simulink model "MCLV_V2_33EP256MC506_SlidingModeObserver_Single_DualShunt"  (R2015b)
settings: Solver=FixedStepDiscrete  StartTime=0.0  StopTime=10.0  FixedStep=.00005  RelTol=1e-3
PreLoadFcn:
  | UserParams;
values from neighbouring files (symbols this model uses):
  DELTA_STARTUP_RAMP = round( (MINSPEEDINRPM*POLEPAIRS*LOOPTIMEINSEC*LOOPTIMEINSEC*65536*65536/(60*OPENLOOPTIMEINSEC)) )    [UserParams.m]
  TS = LOOPTIMEINSEC    (= 5e-05)    [UserParams.m]
undefined symbols (not defined in the file or in its folder): A4, C5, DiscIntNeverNeededParam, F1, Max, ms, P20, P53, P97, Pin, PWMmax, Resol, Timer, us
libraries: MCHP_Blockset x15, simulink x10, Lib_MCHP_BLKDEMO_Motor x2
settings Model: Creator=M91449  LastModifiedBy=M91449
settings OptimizationCC: DefaultParameterBehavior=Inlined  OptimizeModelRefInitCode=on  LifeSpan=1
settings HardwareCC: ProdBitPerInt=16  ProdBitPerPointer=32  ProdLargestAtomicInteger=Integer  ProdLargestAtomicFloat=None  ProdWordSize=16  ProdHWDeviceType=Generic->Custom
settings ModelReferenceCC: ModelReferenceNumInstancesAllowed=Single
settings RTWCC: SystemTargetFile=MCHP_dsPIC_stf.tlc  TemplateMakefile=MCHP_dsPIC.tmf  Description=Microchip Embedded Target PIC24 dsPIC30 dsPIC33 (real-time)  GenerateReport=on  IncludeHyperlinkInReport=on  LaunchReport=on  GenerateTraceInfo=on  GenerateTraceReport=on  GenerateTraceReportSl=on  GenerateTraceReportSf=on  GenerateTraceReportEml=on
settings CodeAppCC: IgnoreCustomStorageClasses=off  MaxIdLength=255
settings STFCustomTargetCC: TargetLibSuffix=_lib.a  ConcurrentExecutionCompliant=off  IncludeMdlTerminateFcn=off  GeneratePreprocessorConditionals=Use local settings  CombineOutputUpdateFcns=on  SuppressErrorStatus=on  ERTCustomFileBanners=on  SupportContinuousTime=off  MATLABClassNameForMDSCustomization=Simulink.SoftwareTarget.ERTCustomization  CPPClassGenCompliant=off  GRTInterface=off  SystemTargetFile=MCHP_dsPIC_stf.tlc
settings ERTTargetCC: TargetLibSuffix=_lib.a  ParMdlRefBuildCompliant=off  CompOptLevelCompliant=off  ConcurrentExecutionCompliant=off  IncludeMdlTerminateFcn=off  SuppressErrorStatus=on  ERTFirstTimeCompliant=off  SupportNonInlinedSFcns=on  ModelStepFunctionPrototypeControlCompliant=off  CPPClassGenCompliant=off  UseToolchainInfoCompliant=off  InlinedParameterPlacement=NonHierarchical  ERTSrcFileBannerTemplate=MCHP_dsPIC_code_template.cgt  ERTHdrFileBannerTemplate=MCHP_dsPIC_code_template.cgt  ERTDataSrcFileTemplate=MCHP_dsPIC_code_template.cgt  ERTDataHdrFileTemplate=MCHP_dsPIC_code_template.cgt  ERTCustomFileTemplate=MCHP_main.tlc

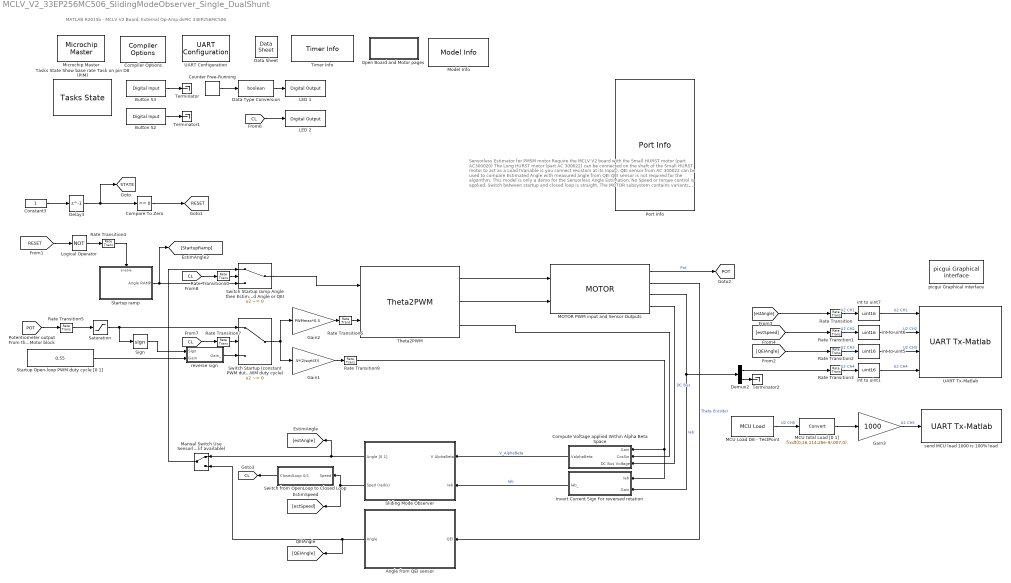
== system MCLV_V2_33EP256MC506_SlidingModeObserver_Single_DualShunt ==
  note: MATLAB R2015b - MCLV V2 Board, External Op-Amp dsPIC 33EP256MC506
  note: Sensorless Estimator for PMSM motor
      | Require the MCLV V2 board with the Small HURST motor (part AC300020)
      | The Long HURST motor (part AC 300022) can be connected on the shaft of the Small HURST motor
      | to act as a Load (Variable is you connect resistors at its Input).
      | QEI sensor from AC 300022 can be used to compare Estimated Angle with measured angle from QEI
      | QEI sensor is not required for the algorithm.
      |
      | This model is only a demo for the Sensorless Angle Estimation.
      | No Speed or torque control is applied. Switch between startup and closed loop is straight.
      |
      | The MOTOR subsystem contains variants. Right click on that MOTOR, and select
      | Dual Shunt or Single Shunt (edge aligned or center aligned) variants.
      | You might have to update the model twice after selecting a different variant.
      |
      | The Potentiometer were saturated to positive value only
      | as negative values does not work with Single Shunt Center Aligned for now
      |
      | MCU load is within 50% and 60% depending on Motor Variant selected.
      | Speed/Torque control loop might be executed at a lower rate than the model base rate (10kHz).
  Angle from QEI sensor : Subsystem
  Button S2 : MCHP_Blockset/Digital IO/Digital Input  PORT=Dynamic Options  PORT_TXT="G   [ 6 : 9 ]"  PIN=7  PACK=off  SIMULTANEOUS=off  ORDERING=None  SampleTime=.1  MCHP_PORT={Digital In}{DIN}2:0:G7;  MCHP_MASTERLINK=MCLV_V2_33EP256MC506_SlidingModeObserver_Single_DualShunt/Microchip Master
  Button S3 : MCHP_Blockset/Digital IO/Digital Input  PORT=Dynamic Options  PORT_TXT="G   [ 6 : 9 ]"  PIN=6  PACK=off  SIMULTANEOUS=off  ORDERING=None  SampleTime=.1  MCHP_PORT={Digital In}{DIN}2:0:G6;  MCHP_MASTERLINK=MCLV_V2_33EP256MC506_SlidingModeObserver_Single_DualShunt/Microchip Master
  Compare To Zero : simulink/Logic and Bit Operations/Compare To Zero  relop===  OutDataTypeStr=boolean
  Compiler Options : MCHP_Blockset/System Configuration/Compiler Options  Priority=1  LATEST_CMPLR=on  COMP_LIST=Dynamic Options  COMP_LIST_TXT=xc16 - v1.26  USE_64BIT_DOUBLE=off  MCHP_MULTITHREAD_COMPILATION=on  MCHP_MASTERLINK=MCLV_V2_33EP256MC506_SlidingModeObserver_Single_DualShunt/Microchip Master  OPTIMIZATION_LEVEL=3  MPLAB_LINKLIB=default  MPLAB_LINKLIB1=default  UNROLL_LOOPS=on  OMIT_FRAME_POINTER=off  PROCEDURAL_ABSTRACTION=off  MCONST=in code memory  MDATA=Use only memory below address 8192 (faster)  MSCALAR=Use only memory below address 8192 (faster)  MCODE=is less than 32768 (faster)  HEAP_SIZE=0  OMF=elf  DEBUG_INFO=off  AssemblyListing=on  ProduceHexOutput=off
  Compute Voltage applied Within Alpha Beta Space : Subsystem
  Constant3 : Constant  OutDataTypeStr=uint16  SampleTime=.1
  Counter Free-Running : simulink/Sources/Counter Free-Running  NumBits=1  tsamp=.1
  Data Sheet : MCHP_Blockset/System Info/Data Sheet  DOC_Type=datasheet  DOC_MCHP_Id=33EP256MC506_datasheet  DOC_FilePath=C:\Users\M91449\AppData\Local\Temp\70000657H.pdf  DOC_FileLastCheckTime="[2016              1             28             13             25         44.133]"  cpy_MCHP_Id=33EP256MC506  MCHP_MASTERLINK=MCLV_V2_33EP256MC506_SlidingModeObserver_Single_DualShunt/Microchip Master
      settings: AttributesFormatString=%<cpy_MCHP_Id>
  Data Type Conversion : DataTypeConversion  OutDataTypeStr=boolean
  Delay3 : Delay  DelayLength=1  InitialCondition=0
  Demux2 : Demux  Outputs=2
  Gain1 : Gain  Gain=.5*(2/sqrt(3))  OutDataTypeStr=fixdt(1,16,15)
  Gain2 : Gain  Gain=PWMmax*0.5  OutMin=-PWMmax*0.5  OutMax=PWMmax*0.5  OutDataTypeStr=fixdt(1,16)
  Gain3 : Gain  Gain=1000  OutDataTypeStr=uint16
  Invert Current Sign For reversed rotation : Subsystem
  LED 1 : MCHP_Blockset/Digital IO/Digital Output  PORT=Dynamic Options  PORT_TXT="D   [ 5  6  8 ]"  PIN=6  PACK=off  SIMULTANEOUS=off  READPREVIOUS=off  ORDERING=None  SampleTime=-1  MCHP_MASTERLINK=MCLV_V2_33EP256MC506_SlidingModeObserver_Single_DualShunt/Microchip Master
  LED 2 : MCHP_Blockset/Digital IO/Digital Output  PORT=Dynamic Options  PORT_TXT="D   [ 5  6  8 ]"  PIN=5  PACK=off  SIMULTANEOUS=off  READPREVIOUS=off  ORDERING=None  SampleTime=-1  MCHP_MASTERLINK=MCLV_V2_33EP256MC506_SlidingModeObserver_Single_DualShunt/Microchip Master
  Logical Operator : Logic  Operator=NOT  AllPortsSameDT=off  OutDataTypeStr=boolean
  MCU Load D8 - TestPoint : MCHP_Blockset/Profiling/MCU Load  MCULoadPin=Dynamic Options  MCULoadPin_TXT=None  MCULoadMeasure=on  TIMER_Resolution=Dynamic Options  TIMER_Resolution_TXT="Resol: 0.1143(us)  -  Max: 7.49(ms)"  MCHP_TIMER_REQUEST={MCU_Load}{MCU_Load}21:5:0:0:[]:524288;  MCHP_TIMER_RESULT=[2 65535 ]  MCHP_MASTERLINK=MCLV_V2_33EP256MC506_SlidingModeObserver_Single_DualShunt/Microchip Master  MCHP_COMPILED_INFO="CompiledSampleTime= [0.0070000000000000001   0 ];CompiledInportDataTypes=[ ];CompiledInportDataWidth=[];"  Info="Timer 2:  Resol: 114.2857143(ns)  -  Max: 7.48983(ms)"  SampleTime=.007
  MCU total Load [0 1] : DataTypeConversion  OutDataTypeStr=fixdt(0,16,114.28e-9/.007,0)  ConvertRealWorld=Stored Integer (SI)
  MOTOR PWM input and Sensor Outputs : Lib_MCHP_BLKDEMO_Motor/MOTOR  OverrideUsingVariant=(default)
  Manual Switch Use Sensorless Estimation or QEI (if available) : ManualSwitch
  Microchip Master : MCHP_Blockset/System Configuration/Microchip Master  Priority=1  PICREF=33EP256MC506  TIMESTEP_REF="Timer  ( 5e-05s )"  BUSYFLAG=Dynamic Options  BUSYFLAG_TXT=None  PWRTEN=PWRT enabled  BOREN=Disable  BODENV=2.7V  BORV=Brown-out Reset set at 2.0V  FPWRT=128ms  DSBOREN=Deep Sleep BOR enabled in Deep Sleep  DSLPBOR=Deep Sleep BOR enabled in Deep Sleep  MCLRE=RA5 input pin disabled;MCLR pin enabled  SMCLR=MCLR pin generates a normal system Reset  PMDL1WAY=Allow only one reconfiguration  RSTPRI=Device will obtain reset instruction from Primary flash  TEMP=Not used  SOSCSRC=Analog Mode for use with crystal  SOSCSEL=Secondary oscillator configured for high-power operation  IOL1WAY=Allow only one reconfiguration  ALTVREF=Voltage reference input; ADC =RA9/RA10 Comparator =RA9;RA10  DISUVREG=Regulator is disabled  DSSWEN=Deep Sleep is controlled by the register bit DSEN  LPCFG=Disabled - regardless of RETEN  RTCBAT=RTC operation is continued through VBAT  VBTBOR=VBAT BOR enabled  WUTSEL=Default regulator start-up time used  POWERSAVE=off  FNOSC=Primary oscillator (XT; HS; EC)  FPR=ECIO w/ PLL 16x  FOSFPR=HS3 w/PLL 16x  FOS=Primary Oscillator  FRANGE=High Range  OSCILLATOR_SELECT=Crystal / Ceramic resonator  OSCILLATOR_SELECT_spd=Crystal / Ceramic resonator  QUARTZ=8e6  QUARTZ_spd=8e6  POSCGAIN=2x gain setting  POSCBOOST=Boost the kick start of the oscillator  SOSCGAIN=2x gain setting  SOSCBOOST=Boost the kick start of the oscillator  ACTIV_PLL=on  ACTIV_PLL_spd=on  MIPS_DESIRED=70e6  MIPS_DESIRED_spd=70e6  FPLLMUL=24x Multiplier  FPLLIDIV=8x Divider  POSCFREQ=Primary oscillator/external clock input frequency greater than 8MHz  POSCMD=XT Crystal Oscillator Mode  POSCMOD=Primary Oscillator Disabled  MIPS=70 * 1e6  FPLLODIV=32x Divider  PLLKEN=Clock switch to PLL source will wait until the PLL lock signal is valid.  FCKSM=Both Clock Switching and Fail-safe Clock Monitor are enabled  FCKSMEN=Sw Disabled; Mon Disabled  IESO=Start up with FRC; then switch  DSWDTPS=1:2;147;483;648 (25.7 Days)  FWDTEN=Disable  FWDTWINSZ=Window size is 25%  FWPSA=WDT prescaler ratio of 1:128  FWPSA0=1:128  FWPSB=1:16  WDT=Disable  WDTPOST=1:32768  WDTPRE=1:128  WDTPS=1:32768  WINDIS=Watchdog Timer in Non-Window mode  WWDTEN=Non-Window mode  DSWDTEN=DSWDT enabled  DSWDTOSC=DSWDT uses Low Power RC Oscillator (LPRC)  FPBDIV=Pb_Clk is Sys_Clk/8  FSOSCEN=Enable SOSC  LPRCSEL=High Power; High Accuracy Mode  OSCIOFCN=OSCO/CLKO/RC15 functions as CLKO (FOSC/2)  OSCIOFNC=OSC2 is clock output  LVRCFG=Low Voltage regulator is not available  PLL_96MHZ=Enabled  PLL96MHZ=96 MHz PLL Startup is enabled automatically on start-up  PLLDIV=PLL is disabled  WDTCLK=WDT uses LPRC  WDTCMX=WDT clock source is determined by the WDTCLK Configuration bits  WDTWIN=WDT Window is 25% of WDT period  APL=Aux Flash Code protect is disabled  APLK=Aux Flash Write Protection or Code Protection is Enabled  AWRP=Auxiliary program memory is not write-protected  BSS=No boot program Flash segment  BWP=Protection Disabled  BWRP=Boot Segment may be written  CP=Protection Disabled  EBS=No Boot EEPROM  ESS=No Segment Data EEPROM  GCP=General Segment Code protect is disabled  GSS=General Segment Code protect is disabled  GSS0=No protection  GSSK=General Segment Write Protection or Code Protection is Enabled  GWRP=General Segment may be written  PWP=Disable  RBS=No Boot RAM  RSS=No Secure RAM  SSS=No Secure Segment  SWRP=Secure segment may be written  WPCFG=Disable  WPDIS=Disable  WPEND=Write Protect from WPFP to the last page of memory  WPFP=Page 127 (0x1FC00)  ICESEL=Communicate on PGEC1/PGED1  ICS=Communicate on PGEC2 and PGED2  JTAGEN=Disable  COE=Reset Into Operational Mode  RES=Not used  DEBUG=Debugger is disabled  BACKBUG=Not used  BKBUG=Device resets into Operational mode  ALTI2C=I2C mapped to SDA1/SCL1 pins  ALTI2C1=I2C1 mapped to SDA1/SCL1 pins  ALTI2C2=I2C2 mapped to SDA2/SCL2 pins  ALTQIO=QEA1; QEB1; INDX1 are selected as inputs to QEI1  ALTSS1=SS1A is selected as the I/O pin for SPI1  CMPPOL0=Hysteresis is applied to falling edge  CMPPOL1=Hysteresis is applied to falling edge  FCANIO=Default CAN I/O  FETHIO=Default Ethernet I/O  FMIIEN=MII Enabled  FSRSSEL=SRS Priority 7  FUSBIDIO=Controlled by the USB Module  FVBUSONIO=Controlled by USB Module  HPOL=PWM module high side output pins have active-high output polarity  HYST0=45 mV Hysteresis  HYST1=45 mV Hysteresis  I2C1SEL=Use Default SCL1/SDA1 Pins For I2C1  LPOL=PWM module low side output pins have active-high output polarity  PWMPIN=PWM module pins controlled by PORT register at device Reset  RTCOSC=RTCC uses Secondary Oscillator (SOSC)  UPLLEN=USB PLL is enabled  UPLLIDIV=12x Divider  ATMOD8=Not used  ALTPMP=EPMP pins are in default location mode  I2C2SEL=I2C2 is multiplexed to SDA2/RA3 and SCL2/RA2  ALTADREF=AVREF+/AVREF- are mapped to RA9/RA10  ALTCVREF=CVREF+/CVREF- are mapped to RA9/RA10  PWMLOCK=PWM registers may be written without key sequence  MCHP_TIMER_REQUEST={Time Step}{TS}0:2:3:1:[]:3500;  MCHP_TIMER_RESULT=[1 3498.9999999999991 ]  MCHP_PLLRegisters="[5    243  16385     -1]"  MCHPVAR=MCHP.fcy.periph=70000000;MCHP.fcy.MIPS=70000000;MCHP.PowerSave=0;MCHP.TimeStepFactor=MCHP_Fun.Hex2num('[3FF0000000000001]');MCHP.TimeStep_Timer=1;MCHP.NTIMERS=5;MCHP.id.name='33EP256MC506';MCHP.id.N=reshape([33 256 506],1,3);MCHP.id.L=reshape({ 'EP','MC',''},1,3);MCHP.id.Arch=3;MCHP.periph.PPS.reg_RPINRx=reshape([-1 1 1 -1 -1 -1 1 -1 -1 -1 -1 -1 -1 -1 1 1 1 1 -1 -1 -1 -1 -1 -1 1 1 -1 -1 1 1 1 1 -1 -1 -1 -1 1 -1 1 -1 -1 -1 -1 -1 1 1 1 -1 -1 -1 -1 -1 1 -1 -1 -1 -1 -1 -1 -1 -1 -1 -1 -1 -1 -1 -1 -1 -1 -1 -1 -1 -1 -1 -1 1 -1 1 1 1],1,80);MCHP.PPS.dsPIC.RP=reshape([-1 -1 -1 -1 -1 -1 -1 -1 -1 -1 -1 -1 -1 -1 -1 -1 -1 -1 -1 -1 4 -1 -1 -1 -1 -1 -1 -1 -1 -1 -1 -1 -1 -1 -1 19 20 21 22 23 24 25 26 27 -1 -1 -1 -1 -1 -1 -1 -1 -1 -1 38 39 40 41 -1 -1 -1 -1 -1 -1 -1 -1 -1 -1 -1 -1 -1 -1 -1 -1 -1 -1 -1 -1 -1 -1 -1 -1 -1 -1 -1 -1 -1 -1 -1 -1 -1 -1 -1 -1 -1 -1 -1 81 -1 -1 -1 -1 -1 -1 -1 -1 -1 -1 -1 -1 -1 -1 -1 -1 -1 -1 -1 -1 102 -1 104],1,121);MCHP.PPS.dsPIC.RPI=reshape([-1 -1 -1 -1 -1 -1 -1 -1 -1 -1 -1 -1 -1 -1 -1 -1 -1 -1 -1 -1 -1 -1 -1 -1 8 9 -1 11 12 -1 -1 -1 16 17 18 -1 -1 -1 -1 -1 -1 -1 -1 -1 28 29 30 31 -1 -1 -1 35 36 37 -1 -1 -1 -1 42 -1 -1 -1 -1 -1 -1 -1 -1 -1 -1 -1 -1 -1 -1 -1 -1 -1 -1 -1 -1 -1 -1 -1 -1 -1 -1 -1 -1 -1 -1 -1 -1 -1 -1 -1 78 79 80 -1 -1 -1 -1 -1 -1 -1 -1 -1 -1 -1 -1 -1 -1 -1 -1 -1 -1 -1 -1 -1 -1 103 -1 105],1,122);MCHP.PPS.dsPIC.RPINR_list=reshape({ '1','INT1','INT2','INT3','INT4','T1CK','T2CK','T3CK','T4CK','T5CK','T6CK','T7CK','T8CK','T9CK','IC1','IC2','IC3','IC4','IC5','IC6','IC7','IC8','OCFA','OCFB','FLT1','FLT2','FLT3','FLT4','QEA1','QEB1','INDX1','HOME1','QEA2','QEB2','INDX2','HOME2','U1RX','U1CTS','U2RX','U2CTS','SDI1','SCK1','SS1','44','SDI2','SCK2','SS2','48','CSDIR','CSCK','COFS','52','C1RX','C2RX','U3RX','U3CTS','U4RX','U4CTS','SDI3','SCK3','SS3','62','SDI4','SCK4','SS4','66','IC9','IC10','IC11','IC12','IC13','IC14','IC15','IC16','OCFC','SYNCI1','SYNCI2','DTCMP1','DTCMP2','DTCMP3','DTCMP4','DTCMP5','DTCMP6','DTCMP7','FLT5','FLT6','FLT7','FLT8','89','SENT1','SENT2','92'},1,92);MCHP.PPS.dsPIC.RPOR_list=reshape({ '1','U1TX','U1RTS','U2TX','U2RTS','SDO1','SCK1','SS1','SDO2','SCK2','SS2','CSDO','CSCK','COFS','C1TX','C2TX','OC1','OC2','OC3','OC4','OC5','OC6','OC7','OC8','C1OUT','C2OUT','C3OUT','U3TX','U3RTS','U4TX','U4RTS','SDO3','SCK3','SS3','SDO4','SCK4','SS4','OC9','OC10','OC11','OC12','OC13','OC14','OC15','OC16','SYNCO1','SYNCO2','QEI1CCMP','QEI2CCMP','REFCLK','C4OUT','C5OUT','52','53','54','55','56','SENT1','SENT2'},1,59);MCHP.PPS.map_RPnR_RPORx=reshape([20 35 36 37 38 39 40 41 42 43 54 55 56 57 -1 97 -1 118 120],1,19);MCHP.Rx=reshape([13 15 21 -1 -1 58 -1 -1 -1 -1 -1 14 16 22 -1 -1 59 -1 -1 -1 -1 -1 -1 17 23 -1 -1 -1 -1 -1 -1 -1 -1 -1 18 35 -1 -1 -1 -1 -1 -1 -1 -1 33 32 36 -1 -1 -1 -1 -1 -1 -1 -1 -1 43 37 53 -1 -1 -1 -1 -1 -1 -1 -1 44 50 54 -1 -1 4 -1 -1 -1 -1 1 46 51 -1 -1 -1 5 -1 -1 -1 -1 31 48 52 42 -1 -1 6 -1 -1 -1 -1 34 49 55 -1 -1 -1 8 -1 -1 -1 -1 64 60 45 -1 -1 -1 -1 -1 -1 -1 -1 12 61 24 -1 -1 -1 -1 -1 -1 -1 -1 11 62 39 -1 27 -1 -1 -1 -1 -1 -1 -1 63 47 -1 28 -1 -1 -1 -1 -1 -1 -1 2 -1 -1 29 -1 -1 -1 -1 -1 -1 -1 3 40 -1 30 -1 -1 -1 -1 -1 -1],11,16);MCHP.ADC.ANtype=reshape([3 0],1,2);MCHP.ADC.ADCONx=reshape([47103 59391 40959 263 0 0],1,6);MCHP.ADC.ADCHS_0=reshape([40863 1799],1,2);MCHP.ADC.Flags=reshape([1 0],1,2);MCHP.ADC.Buffer=reshape([16 -1],1,2);MCHP.ADC.port=reshape([0 1 16 17 18 19 32 33 34 11 12 43 76 77 78 79 -1 -1 -1 -1 -1 -1 -1 -1 -1 -1 -1 -1 -1 -1 -1 -1 -1 -1 -1 -1 -1 -1 -1 -1 -1 -1 -1 -1 -1 -1 -1 -1 -1 -1 -1 -1 -1 -1 -1 -1 -1],1,57);MCHP.ADC.port_VrefP=17;MCHP.ADC.port_VrefM=16;MCHP.ADC.port_AVdd=-1;MCHP.ADC.port_AVss=-1;MCHP.memory.RAM=32768;MCHP.memory.RAM_XBegin=4096;MCHP.memory.RAM_YBegin=20480;MCHP.memory.RAM_dma=reshape([-1 -1],1,2);MCHP.DMA.Num=4;MCHP.DMA.CNTmax=16383;MCHP.QEI.QEICONx=reshape([49023 -1 -1 -1 -1 -1],1,6);MCHP.QEI.QEItype=1;MCHP.QEI.Port_QEI_INDX=reshape([-1 -1],1,2);MCHP.QEI.Port_QEI_QEA=reshape([-1 -1],1,2);MCHP.QEI.Port_QEI_QEB=reshape([-1 -1],1,2);MCHP.QEI.Port_QEI_UPDN=reshape([-1 -1],1,2);MCHP.INT.Port=reshape([23 32767 32767 -1 -1],1,5);MCHP.PWM_HS.Flags=reshape([3 1 0],1,3);MCHP.PWM.port_FLT=reshape([-1 -1 -1 34 43 -1 -1 -1 -1 -1 -1 -1 -1 -1 -1 -1 -1 -1 -1 -1 -1 -1 -1 -1 -1 -1 -1 -1 -1 -1 -1 -1 20],1,33);MCHP.PWM.PWMRef=-1;MCHP.PWM.Flag=0;MCHP.PWM.Port_PWM_l=reshape([31 -1 29 -1 27 -1 -1 -1 -1 -1 -1 -1 -1 -1 -1 -1 -1 -1],2,9);MCHP.PWM.Port_PWM_h=reshape([30 -1 28 -1 26 -1 -1 -1 -1 -1 -1 -1 -1 -1 -1 -1 -1 -1],2,9);MCHP.IC.Port=reshape([32767 32767 32767 32767 0 0 0 0 0 0 0 0 0 0 0 0],1,16);MCHP.IC.type=1;MCHP.OC.Port=reshape([32767 32767 32767 32767 0 0 0 0 0 0 0 0 0 0 0 0],1,16);MCHP.OC.type=1;MCHP.CN.Port=reshape([-1 -1 -1 -1 -1 -1 -1 -1 -1 -1 -1 -1 -1 -1 -1 -1 -1 -1 -1 -1 -1 -1 -1 -1 -1 -1 -1 -1 -1 -1 -1 -1 -1 -1 -1 -1 -1 -1 -1 -1 -1 -1 -1 -1 -1 -1 -1 -1 -1 -1 -1 -1 -1 -1 -1 -1 -1 -1 -1 -1 -1 -1 -1 -1 -1 -1 -1 -1 -1 -1 -1 -1 -1 -1 -1 -1 -1 -1 -1 -1 -1 -1 -1 -1 -1],1,85);MCHP.CN.PullUp=reshape([8083 65535 49151 352 61440 3 960 0 0 0 0],1,11);MCHP.CN.type=1;MCHP.CN.Flag_PullDown=1;MCHP.SPI.Refs=reshape([1 2 0 0 0 0],1,6);MCHP.SPI.SPIxCON1=8191;MCHP.SPI.SPIxCON2=57347;MCHP.SPI.Port_SDI=reshape([9 -1 -1 -1 -1 -1],1,6);MCHP.SPI.Port_SDO=reshape([4 -1 -1 -1 -1 -1],1,6);MCHP.SPI.Port_SCK=reshape([35 -1 -1 -1 -1 -1],1,6);MCHP.SPI.Port_SS=reshape([16 -1 -1 -1 -1 -1],1,6);MCHP.I2C.Refs=reshape([1 2 0 0 0],1,5);MCHP.I2C.I2CxCON=49151;MCHP.I2C.NewRegName=1;MCHP.I2C.Port_SDA=reshape([36 8 -1 -1 -1],1,5);MCHP.I2C.Port_SCL=reshape([37 20 -1 -1 -1],1,5);MCHP.I2C.Port_ASDA=reshape([25 21 -1 -1 -1],1,5);MCHP.I2C.Port_ASCL=reshape([24 22 -1 -1 -1],1,5);MCHP.I2C.Fuse_Port_SCL_SDA=reshape([3 1 4 1 -1 -1 -1 -1 -1 -1],2,5);MCHP.I2C.Fuse_Port_ASCL_ASDA=reshape([3 2 4 2 -1 -1 -1 -1 -1 -1],2,5);MCHP.Comp.Port_CVrefin=-1;MCHP.Comp.Port_CVref=-1;MCHP.Comp.Port_CVref1O=24;MCHP.Comp.Port_CVref2O=4;MCHP.Comp.Port_CxOUT=reshape([32767 32767 32767 32767 -1],1,5);MCHP.Comp.Port_OAxOUT=reshape([17 0 32 -1 -1],1,5);MCHP.Comp.Port_CxINP=reshape([18 1 34 32 -1],1,5);MCHP.Comp.Port_CxINM=reshape([19 43 -1 -1 16 76 -1 -1 33 77 -1 -1 33 -1 -1 -1 -1 -1 -1 -1],4,5);MCHP.Comp.nComp=reshape([4 0 0],1,3);MCHP.Comp.OpAmp=7;MCHP.Comp.CVRCON=reshape([17663 0],1,2);MCHP.UART.port_Rx=reshape([32767 32767 -1 -1 -1 -1],1,6);MCHP.UART.port_Tx=reshape([32767 32767 -1 -1 -1 -1],1,6);MCHP.UART.port_ARx=reshape([-1 -1],1,2);MCHP.UART.port_ATx=reshape([-1 -1],1,2);MCHP.UART.port_RTS=reshape([34 76 -1 -1 -1 -1],1,6);MCHP.UART.port_CTS=reshape([43 77 -1 -1 -1 -1],1,6);MCHP.UART.reg_UxMODE=reshape([48127 48127 -1 -1 -1 -1],1,6);MCHP.UART.reg_UxSTA=reshape([61439 61439 -1 -1 -1 -1],1,6);  MCHP_CRC=2647204  BTMODE=Device is in Single Boot (legacy) mode  RES1=Not used  PLLSS=PLL is fed by the Primary oscillator  RES2=Not used  ALTCMPI=C1INC is on RB13; C2INC is on RB9 and C3INC is on RA0  BOREN1=BOR Enabled [When BOREN=1]  ALTRB6=Append the RP6/ASCL1/PMPD6 functions of RB6 to RA1 pin functions  RETCFG=Retention regulator is not available  DFMCY=Not used  BSS2=No Boot Segment  BSEN=No Boot Segment  CWRP=Configuration Segment may be written  CSS=No Protection (other than CWRP)  AIVTDIS=Disable Alternate Vector Table  BSLIM=Not used  WDTEN=Disable  BTSWP=Not used  DBCC=Not used  CTXT1=Not Assigned  CTXT2=Not Assigned  SEQNUM=Not used  nSEQNUM=Not used  BOREN0=Enabled  DMTIVT=Not used  DMTCNT=2^31 (2147483648)  DMTEN=Dead Man Timer is Disabled and can be enabled by software  ON=Not used  USERID=Not used  RESERVED1=Not used  PGL1WAY=Allow only one reconfiguration  FPLLRNG=34-68 MHz Input  FPLLICLK=FRC is input to the System PLL  FPLLMULT=PLL Multiply by 128  UPLLFSEL=USB PLL input is 24 MHz  DMTINTV=Window/Interval value is 127/128 counter value  WDTSPGM=WDT stops during Flash programming  FDMTEN=Deadman Timer is disabled  TRCEN=Trace features in the CPU are enabled  BOOTISA=Boot code and Exception code is MIPS32  FECCCON=ECC and Dynamic ECC are disabled (ECCCON bits are writable)  EXTDDRSIZE=External DDR2 Size is 128 MB  FSLEEP=Flash is powered down when the device is in Sleep mode  DBGPER=Allow CPU access to all permission regions  EJTAGBEN=Normal EJTAG functionality  TSEQ=Not used  CSEQ=Not used
  Model Info : simulink/Model-Wide Utilities/Model Info  Frame=on  DisplayStringWithTags=|  HorizontalTextAlignment=Left  LeftAlignmentValue=0.02  SourceBlockDiagram=MCLV_V2_33EP256MC506_SlidingModeObserver_Single_DualShunt  TagMaxNumber=20
      | Short hust motor with:
      | M1 - Black
      | M2 - Red
      | M3 - White
  Open Board and Motor pages : Subsystem
      settings: OpenFcn=|
      | web('www.microchip.com/DevelopmentTools/ProductDetails.aspx?PartNO=DM330021-2','-browser');
      | pause(1);
      | web('http://www.microchipdirect.com/productsearch.aspx?keywords=AC300020','-browser');
      | pause(1);
      | web('www.microchipdirect.com/ProductSearch.aspx?keywords=AC300022','-browser');
      mask Display: disp('Open tools\nWebpage');
  Port Info : MCHP_Blockset/System Info/Port Info  MCHP_MASTERLINK=MCLV_V2_33EP256MC506_SlidingModeObserver_Single_DualShunt/Microchip Master
  Rate Transition{,1..4,6..7,9..10} (9 alike) : RateTransition
  Rate Transition5 : RateTransition  OutPortSampleTime=.1
  Saturation : Saturate  UpperLimit=1  LowerLimit=0
  Sign : Signum
  Sliding Mode Observer : Subsystem
  Startup Open-loop PWM duty cycle [0 1] : Constant  Value=0.55  OutDataTypeStr=Inherit: Inherit via back propagation
  Startup ramp : Subsystem
  Switch Startup (constant PWM duty cycle) then Closed Loop (Pot drive PWM duty cycle) : Switch  Criteria=u2 ~= 0  Threshold=250
  Switch Startup ramp Angle then Estimated Angle or QEI : Switch  Criteria=u2 ~= 0  Threshold=250
  Switch from OpenLoop to Closed Loop : Subsystem
  Tasks State Show base rate Task on pin D8 (PIM) : MCHP_Blockset/Profiling/Tasks State  TasksPin=D8  MCHP_PORT={Task D1 Running}{Task D1}15:1:D8;  MCHP_MASTERLINK=MCLV_V2_33EP256MC506_SlidingModeObserver_Single_DualShunt/Microchip Master
  Terminator : Terminator
  Terminator1 : Terminator
  Terminator2 : Terminator
  Theta2PWM : Lib_MCHP_BLKDEMO_Motor/Theta2PWM  VariantControl=Variant  OverrideUsingVariant=Optimized
  Timer Info : MCHP_Blockset/System Info/Timer Info  MCHP_MASTERLINK=MCLV_V2_33EP256MC506_SlidingModeObserver_Single_DualShunt/Microchip Master
  UART Configuration : MCHP_Blockset/BUS UART/UART Configuration  UART_REF=2  BAUD_Choice=Dynamic Options  BAUD_Choice_TXT="921600         [-0.06%]"  BAUD_Choice_IR=Dynamic Options  BAUD_Choice_IR_TXT=[]  BAUD_Custom=115200  IRDA=off  ALT_IO=on  PIN_RX=Dynamic Options  PIN_RX_TXT=C5 / P53 / Pin[37]  PIN_TX=Dynamic Options  PIN_TX_TXT=F1 / P97 / Pin[59]  FlowControl=None  PIN_CTS=Dynamic Options  PIN_CTS_TXT=A4 / P20 / Pin[33]  PIN_RTS=Dynamic Options  PIN_RTS_TXT=A4 / P20 / Pin[33]  MCHP_PORT="{UART2  Rx}{U2RX}3:0:P53;{UART2  Tx}{U2TX}3:1:P97;"  MCHP_MASTERLINK=MCLV_V2_33EP256MC506_SlidingModeObserver_Single_DualShunt/Microchip Master  MCHP_COM_ExtPil=off  TX_IMPLEMENTATION=DMA Ping-Pong Mode  TX_INT_PRIORITY=2  TX_INT_WHEN=is empty & last char is sent  TX_CIRCULAR_SIZE=32  TX_DMA_CHANNEL="0   (Lowest Priority)"  TX_DMA_SIZE=60  RX_IMPLEMENTATION=Simplest (4 bytes internal buffer only)  RX_INT_PRIORITY=1  RX_INT_WHEN=receive 1 character  RX_CIRCULAR_SIZE=32  InitSequence_chkbox=off  BAUD_Choice_InitSeq=Dynamic Options  BAUD_Choice_InitSeq_TXT="110         [-0.00%]"  BAUD_Choice_IR_InitSeq=Dynamic Options  BAUD_Choice_IR_InitSeq_TXT=0  BAUD_Custom_InitSeq=0  InitSequence='Hello World'
  UART Tx-Matlab : MCHP_Blockset/BUS UART/UART Tx-Matlab  UART_REF=2  CHANNELS=[1 2 3 4]  AllOrNothing=on  SampleTime=.00015  MCHP_MASTERLINK=MCLV_V2_33EP256MC506_SlidingModeObserver_Single_DualShunt/Microchip Master  MCHP_COMPILED_INFO="CompiledSampleTime= [0.00014999999999999999   0 ];CompiledInportDataTypes=[  5   5   5   5 ];CompiledInportDataWidth=[1  1  1  1];"
  int to uint{1,5..7} (4 alike) : DataTypeConversion  OutDataTypeStr=uint16  ConvertRealWorld=Stored Integer (SI)
  picgui Graphical interface : MCHP_Blockset/BUS UART/picgui Graphical interface  Nothing=0
  reverse sign : Subsystem
  send MCU load 1000 is 100% load : MCHP_Blockset/BUS UART/UART Tx-Matlab  UART_REF=2  CHANNELS=5  AllOrNothing=on  SampleTime=-1  MCHP_MASTERLINK=MCLV_V2_33EP256MC506_SlidingModeObserver_Single_DualShunt/Microchip Master  MCHP_COMPILED_INFO="CompiledSampleTime= [0.0070000000000000001   0 ];CompiledInportDataTypes=[  5 ];CompiledInportDataWidth=[1];"
  tag scope: CL=global, POT=global, RESET=global, STATE=global
  wires:
  Counter Free-Running/1 -> Data Type Conversion/1
  Data Type Conversion/1 -> LED 1/1
  [CL] -> LED 2/1
  Rate Transition/1 -> int to uint7/1  "U2 CH1"
  Rate Transition1/1 -> int to uint6/1  "U2 CH2"
  MCU Load D8 - TestPoint/1 -> MCU total Load [0 1]/1  "U2 CH5"
  Constant3/1 -> Delay3/1
  Delay3/1 -> Compare To Zero/1, [STATE]
  Sliding Mode Observer/2(Sped (rad/s)) -> [estSpeed], Switch from OpenLoop to Closed Loop/1(Speed)
  Switch Startup ramp Angle then Estimated Angle or QEI/1 -> Theta2PWM/1
  [estAngle] -> Rate Transition/1
  [estSpeed] -> Rate Transition1/1
  Rate Transition2/1 -> int to uint5/1  "U2 CH3"
  Rate Transition3/1 -> int to uint1/1  "U2 CH4"
  Compare To Zero/1 -> [RESET]
  Theta2PWM/2 -> MOTOR PWM input and Sensor Outputs/2
  Startup ramp/1(Angle RAMP) -> [StartupRamp], Switch Startup ramp Angle then Estimated Angle or QEI/3
  [RESET] -> Logical Operator/1
  Logical Operator/1 -> Rate Transition4/1
  Rate Transition4/1 -> Startup ramp/Enable
  Theta2PWM/1 -> MOTOR PWM input and Sensor Outputs/1
  MOTOR PWM input and Sensor Outputs/3 -> Invert Current Sign For reversed rotation/2(Gain), Demux2/1  "Iab"
  Switch Startup (constant PWM duty cycle) then Closed Loop (Pot drive PWM duty cycle)/1 -> Gain1/1, Gain2/1
  MOTOR PWM input and Sensor Outputs/1 -> [POT]  "Pot"
  [POT] -> Rate Transition5/1
  Rate Transition5/1 -> Saturation/1
  Saturation/1 -> Sign/1, Switch Startup (constant PWM duty cycle) then Closed Loop (Pot drive PWM duty cycle)/1
  Demux2/1 -> Rate Transition3/1
  Manual Switch Use Sensorless Estimation or QEI (if available)/1 -> Switch Startup ramp Angle then Estimated Angle or QEI/1
  int to uint5/1 -> UART Tx-Matlab/3  "U2 CH3"
  [CL] -> Rate Transition7/1
  [CL] -> Rate Transition10/1
  Sliding Mode Observer/1(Angle [0 1]) -> Manual Switch Use Sensorless Estimation or QEI (if available)/1, [estAngle]
  Rate Transition9/1 -> Invert Current Sign For reversed rotation/1(Iab), Compute Voltage applied Within Alpha Beta Space/1(Gain)
  Gain2/1 -> Rate Transition6/1
  Rate Transition6/1 -> Theta2PWM/2
  Gain1/1 -> Rate Transition9/1
  Angle from QEI sensor/1(Angle) -> [QEIAngle], Manual Switch Use Sensorless Estimation or QEI (if available)/2
  MOTOR PWM input and Sensor Outputs/2 -> Angle from QEI sensor/1(QEI)  "Theta Encoder"
  Invert Current Sign For reversed rotation/1("Iab_ ") -> Sliding Mode Observer/2(Iab)  "Iab"
  MOTOR PWM input and Sensor Outputs/4 -> Compute Voltage applied Within Alpha Beta Space/3(DC Bus Voltage)  "DC Bus"
  Theta2PWM/3 -> Compute Voltage applied Within Alpha Beta Space/2(CosSin)
  Compute Voltage applied Within Alpha Beta Space/1(ValphaBeta) -> Sliding Mode Observer/1(V AlphaBeta)  "V_AlphaBeta"
  Rate Transition7/1 -> Switch Startup (constant PWM duty cycle) then Closed Loop (Pot drive PWM duty cycle)/2
  Rate Transition10/1 -> Switch Startup ramp Angle then Estimated Angle or QEI/2
  Switch from OpenLoop to Closed Loop/1(ClosedLoop 0/1) -> [CL]
  reverse sign/1(Gain_) -> Switch Startup (constant PWM duty cycle) then Closed Loop (Pot drive PWM duty cycle)/3
  Sign/1 -> reverse sign/1(Sign)
  Startup Open-loop PWM duty cycle [0 1]/1 -> reverse sign/2(Gain)
  [QEIAngle] -> Rate Transition2/1
  int to uint6/1 -> UART Tx-Matlab/2  "U2 CH2"
  int to uint7/1 -> UART Tx-Matlab/1  "U2 CH1"
  int to uint1/1 -> UART Tx-Matlab/4  "U2 CH4"
  MCU total Load [0 1]/1 -> Gain3/1
  Gain3/1 -> send MCU load 1000 is 100% load/1  "U2 CH5"
  Button S3/1 -> Terminator/1
  Button S2/1 -> Terminator1/1
  Demux2/2 -> Terminator2/1

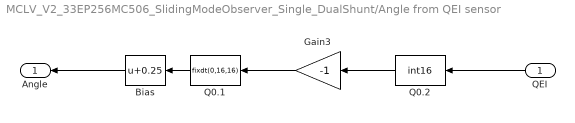
== system MCLV_V2_33EP256MC506_SlidingModeObserver_Single_DualShunt/Angle from QEI sensor ==
  QEI : Inport
  Bias : Bias  Bias=0.25
  Gain3 : Gain  Gain=-1  OutDataTypeStr=Inherit: Same as input
  Q0.1 : DataTypeConversion  OutDataTypeStr=fixdt(0,16,16)  ConvertRealWorld=Stored Integer (SI)
  Q0.2 : DataTypeConversion  OutDataTypeStr=int16  ConvertRealWorld=Stored Integer (SI)
  Angle : Outport
  wires:
  Bias/1 -> Angle/1
  Gain3/1 -> Q0.1/1
  Q0.2/1 -> Gain3/1
  Q0.1/1 -> Bias/1
  QEI/1 -> Q0.2/1

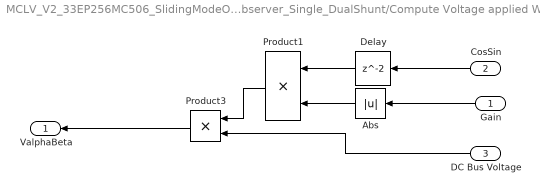
== system MCLV_V2_33EP256MC506_SlidingModeObserver_Single_DualShunt/Compute Voltage applied Within Alpha Beta Space ==
  Gain : Inport
  CosSin : Inport  Port=2
  DC Bus Voltage : Inport  Port=3
  Abs : Abs
  Delay : Delay  InitialCondition=0
  Product1 : Product  OutDataTypeStr=Inherit: Same as first input
  Product3 : Product  OutMin=[-24]  OutMax=[24]  OutDataTypeStr=fixdt(1,16)
  ValphaBeta : Outport
  wires:
  Abs/1 -> Product1/2
  Delay/1 -> Product1/1
  DC Bus Voltage/1 -> Product3/2
  Product1/1 -> Product3/1
  Product3/1 -> ValphaBeta/1
  CosSin/1 -> Delay/1
  Gain/1 -> Abs/1

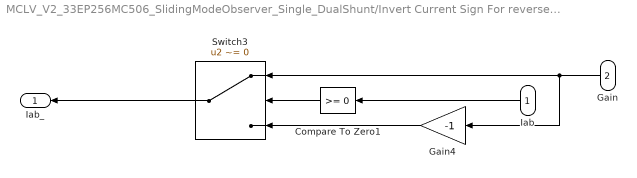
== system MCLV_V2_33EP256MC506_SlidingModeObserver_Single_DualShunt/Invert Current Sign For reversed rotation ==
  Iab : Inport
  Gain : Inport  Port=2
  Compare To Zero1 : simulink/Logic and Bit Operations/Compare To Zero  relop=>=  OutDataTypeStr=boolean
  Gain4 : Gain  Gain=-1  SaturateOnIntegerOverflow=on  OutDataTypeStr=Inherit: Same as input
  Switch3 : Switch  Criteria=u2 ~= 0  Threshold=250
  "Iab_ " : Outport
  wires:
  Gain4/1 -> Switch3/3
  Compare To Zero1/1 -> Switch3/2
  Switch3/1 -> "Iab_ "/1
  Iab/1 -> Compare To Zero1/1
  Gain/1 -> Switch3/1, Gain4/1

== system MCLV_V2_33EP256MC506_SlidingModeObserver_Single_DualShunt/Open Board and Motor pages ==

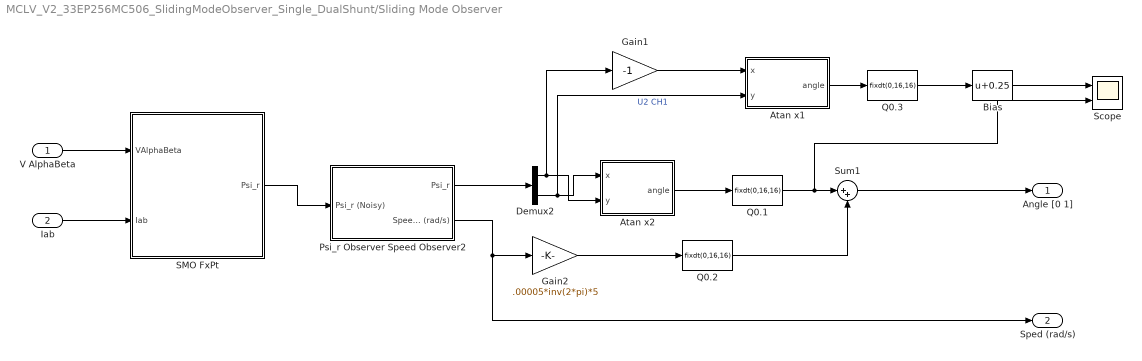
== system MCLV_V2_33EP256MC506_SlidingModeObserver_Single_DualShunt/Sliding Mode Observer ==
  V AlphaBeta : Inport
  Iab : Inport  Port=2
  Atan x1 : Subsystem  AncestorBlock=Lib_MCHP_BLKDEMO_Motor/Atan x2
  Atan x2 : Subsystem  AncestorBlock=Lib_MCHP_BLKDEMO_Motor/Atan x2
  Bias : Bias  Bias=0.25
  Demux2 : Demux  Outputs=2
  Gain1 : Gain  Gain=-1  RndMeth=Simplest  OutDataTypeStr=Inherit: Same as input
  Gain2 : Gain  Gain=.00005*inv(2*pi)*5  OutDataTypeStr=fixdt(1,16,15)  RndMeth=Simplest
  Psi_r Observer Speed Observer2 : Subsystem
  Q0.1 : DataTypeConversion  OutDataTypeStr=fixdt(0,16,16)  ConvertRealWorld=Stored Integer (SI)  RndMeth=Simplest
  Q0.2 : DataTypeConversion  OutDataTypeStr=fixdt(0,16,16)  RndMeth=Simplest
  Q0.3 : DataTypeConversion  OutDataTypeStr=fixdt(0,16,16)  ConvertRealWorld=Stored Integer (SI)  RndMeth=Simplest
  SMO FxPt : Subsystem
  Scope : Scope  NumInputPorts=2
  Sum1 : Sum  Inputs=|++  OutDataTypeStr=Inherit: Same as accumulator  RndMeth=Simplest
  Angle [0 1] : Outport
  Sped (rad/s) : Outport  Port=2
  wires:
  Psi_r Observer Speed Observer2/1(Psi_r) -> Demux2/1
  V AlphaBeta/1 -> SMO FxPt/1(VAlphaBeta)
  Atan x2/1(angle) -> Q0.1/1
  SMO FxPt/1(Psi_r) -> Psi_r Observer Speed Observer2/1(Psi_r (Noisy))
  Psi_r Observer Speed Observer2/2(Speed we (rad/s)) -> Sped (rad/s)/1, Gain2/1
  Iab/1 -> SMO FxPt/2(Iab)
  Sum1/1 -> Angle [0 1]/1
  Q0.1/1 -> Scope/2, Sum1/1
  Demux2/2 -> Atan x1/2(y), Atan x2/1(x)  "U2 CH1"
  Demux2/1 -> Gain1/1, Atan x2/2(y)
  Gain2/1 -> Q0.2/1
  Q0.2/1 -> Sum1/2
  Atan x1/1(angle) -> Q0.3/1
  Gain1/1 -> Atan x1/1(x)
  Q0.3/1 -> Bias/1
  Bias/1 -> Scope/1

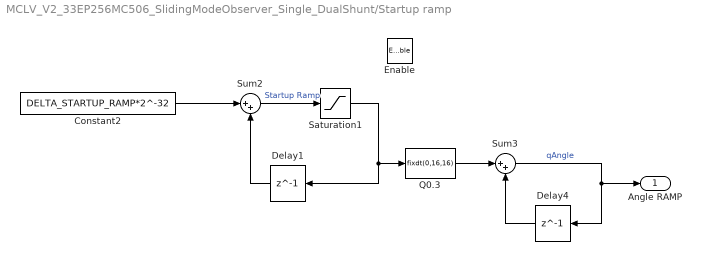
== system MCLV_V2_33EP256MC506_SlidingModeObserver_Single_DualShunt/Startup ramp ==
  Enable : EnablePort  StatesWhenEnabling=reset
  Constant2 : Constant  Value=DELTA_STARTUP_RAMP*2^-32  OutDataTypeStr=fixdt(0,16,32)  SampleTime=.00005
  Delay1 : Delay  DelayLength=1  InitialCondition=0
  Delay4 : Delay  DelayLength=1  InitialCondition=0
  Q0.3 : DataTypeConversion  OutDataTypeStr=fixdt(0,16,16)
  Saturation1 : Saturate  UpperLimit=DELTA_STARTUP_RAMP*2^-32*10/TS  LowerLimit=0
  Sum2 : Sum  Inputs=|++  AccumDataTypeStr=fixdt(0,32,32)  OutDataTypeStr=Inherit: Same as accumulator  RndMeth=Simplest
  Sum3 : Sum  Inputs=|++  AccumDataTypeStr=fixdt(0,16,16)  OutDataTypeStr=Inherit: Same as accumulator  RndMeth=Simplest
  Angle RAMP : Outport
  wires:
  Delay1/1 -> Sum2/2
  Saturation1/1 -> Delay1/1, Q0.3/1
  Sum2/1 -> Saturation1/1  "Startup Ramp"
  Sum3/1 -> Angle RAMP/1, Delay4/1  "qAngle"
  Q0.3/1 -> Sum3/1
  Constant2/1 -> Sum2/1
  Delay4/1 -> Sum3/2

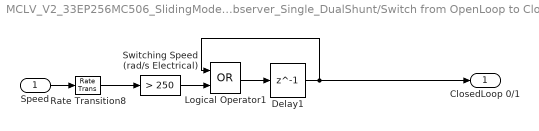
== system MCLV_V2_33EP256MC506_SlidingModeObserver_Single_DualShunt/Switch from OpenLoop to Closed Loop ==
  Speed : Inport
  Delay1 : Delay  DelayLength=1  InitialCondition=[0]
  Logical Operator1 : Logic  Operator=OR  AllPortsSameDT=off  OutDataTypeStr=boolean
  Rate Transition8 : RateTransition  OutPortSampleTime=.01
  Switching Speed (rad/s Electrical) : simulink/Logic and Bit Operations/Compare To Constant  relop=>  const=250  OutDataTypeStr=boolean
  ClosedLoop 0/1 : Outport
  wires:
  Logical Operator1/1 -> Delay1/1
  Switching Speed (rad/s Electrical)/1 -> Logical Operator1/2
  Delay1/1 -> ClosedLoop 0/1/1, Logical Operator1/1
  Rate Transition8/1 -> Switching Speed (rad/s Electrical)/1
  Speed/1 -> Rate Transition8/1

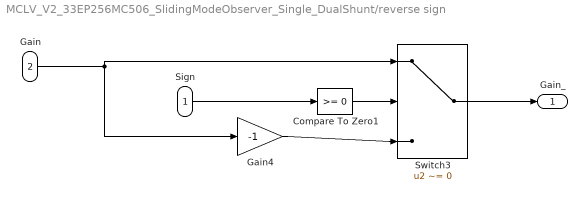
== system MCLV_V2_33EP256MC506_SlidingModeObserver_Single_DualShunt/reverse sign ==
  Sign : Inport
  Gain : Inport  Port=2
  Compare To Zero1 : simulink/Logic and Bit Operations/Compare To Zero  relop=>=  OutDataTypeStr=boolean
  Gain4 : Gain  Gain=-1  SaturateOnIntegerOverflow=on  OutDataTypeStr=Inherit: Same as input
  Switch3 : Switch  Criteria=u2 ~= 0  Threshold=250
  Gain_ : Outport
  wires:
  Sign/1 -> Compare To Zero1/1
  Switch3/1 -> Gain_/1
  Compare To Zero1/1 -> Switch3/2
  Gain4/1 -> Switch3/3
  Gain/1 -> Gain4/1, Switch3/1

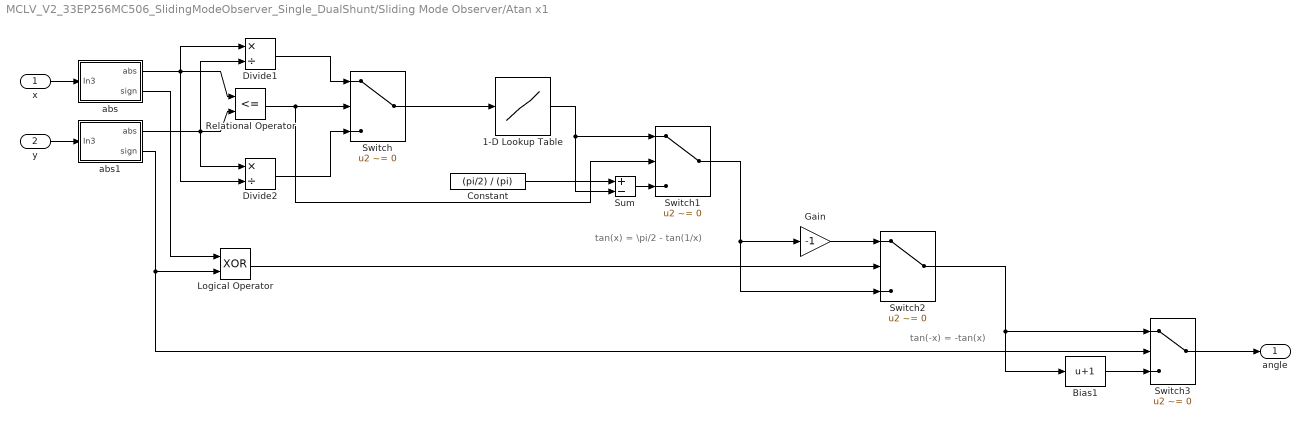
== system MCLV_V2_33EP256MC506_SlidingModeObserver_Single_DualShunt/Sliding Mode Observer/Atan x1 ==
  note: tan(x) = \pi/2 - tan(1/x)
  note: tan(-x) = -tan(x)
  x : Inport
  y : Inport  Port=2
  1-D Lookup Table : Lookup_n-D  NumberOfTableDimensions=1  BreakpointsSpecification=Even spacing  BreakpointsForDimension1=[0:2^-8:1]  BreakpointsForDimension1FirstPoint=0  BreakpointsForDimension1Spacing=2^-8  IndexSearchMethod=Evenly spaced points  BeginIndexSearchUsingPreviousIndexResult=on  Table=atan([0:2^-8:1])/(pi)  TableDataTypeStr=fixdt(1,16,15)  InterpMethod=Flat  ExtrapMethod=Clip  RemoveProtectionInput=on  UseLastTableValue=on  OutDataTypeStr=fixdt(1,16,15)  RndMeth=Simplest  InputSameDT=on  LockScale=on
  Bias1 : Bias  Bias=1
  Constant : Constant  Value=(pi/2) / (pi)  OutDataTypeStr=Inherit: Inherit via back propagation
  Divide1 : Product  Inputs=*/  OutDataTypeStr=fixdt(0,16,15)
  Divide2 : Product  Inputs=*/  OutDataTypeStr=fixdt(0,16,15)
  Gain : Gain  Gain=-1  OutDataTypeStr=Inherit: Same as input
  Logical Operator : Logic  Operator=XOR  AllPortsSameDT=off  OutDataTypeStr=boolean
  Relational Operator : RelationalOperator  Operator=<=  OutDataTypeStr=boolean
  Sum : Sum  Inputs=+-
  Switch{,1..3} (4 alike) : Switch  Criteria=u2 ~= 0
  abs : Subsystem
  abs1 : Subsystem
  angle : Outport
  wires:
  Gain/1 -> Switch2/1
  Bias1/1 -> Switch3/3
  Switch3/1 -> angle/1
  Switch2/1 -> Switch3/1, Bias1/1
  Relational Operator/1 -> Switch/2, Switch1/2
  Divide2/1 -> Switch/3
  Divide1/1 -> Switch/1
  Switch/1 -> 1-D Lookup Table/1
  1-D Lookup Table/1 -> Switch1/1, Sum/2
  Constant/1 -> Sum/1
  Sum/1 -> Switch1/3
  abs/1(abs) -> Relational Operator/1, Divide1/1, Divide2/2
  x/1 -> abs/1(In3)
  abs1/1(abs) -> Relational Operator/2, Divide2/1, Divide1/2
  y/1 -> abs1/1(In3)
  abs/2(sign) -> Logical Operator/1
  abs1/2(sign) -> Logical Operator/2, Switch3/2
  Logical Operator/1 -> Switch2/2
  Switch1/1 -> Gain/1, Switch2/3

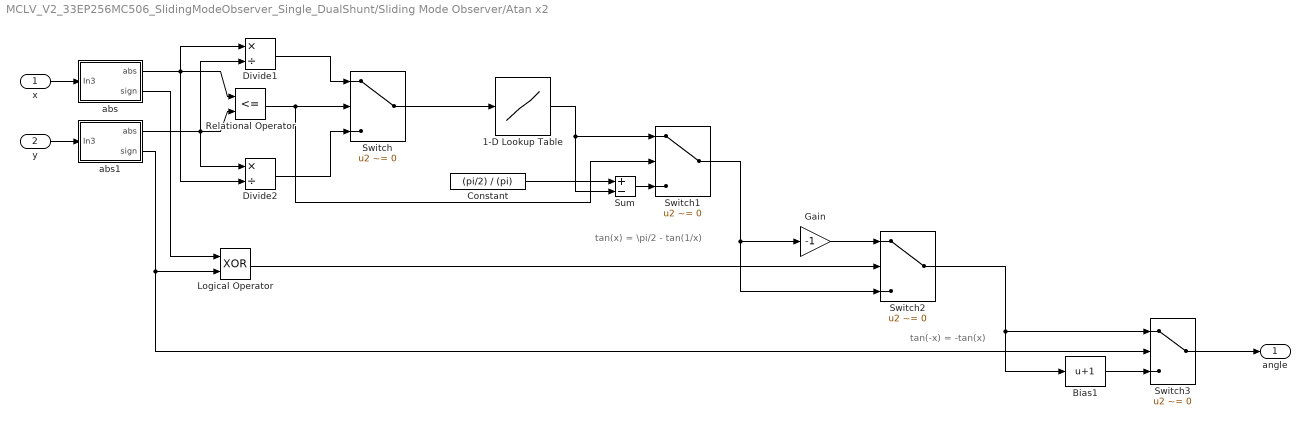
== system MCLV_V2_33EP256MC506_SlidingModeObserver_Single_DualShunt/Sliding Mode Observer/Atan x2 ==
  note: tan(-x) = -tan(x)
  note: tan(x) = \pi/2 - tan(1/x)
  x : Inport
  y : Inport  Port=2
  1-D Lookup Table : Lookup_n-D  NumberOfTableDimensions=1  BreakpointsSpecification=Even spacing  BreakpointsForDimension1=[0:2^-8:1]  BreakpointsForDimension1FirstPoint=0  BreakpointsForDimension1Spacing=2^-8  IndexSearchMethod=Evenly spaced points  BeginIndexSearchUsingPreviousIndexResult=on  Table=atan([0:2^-8:1])/(pi)  TableDataTypeStr=fixdt(1,16,15)  InterpMethod=Flat  ExtrapMethod=Clip  RemoveProtectionInput=on  UseLastTableValue=on  OutDataTypeStr=fixdt(1,16,15)  RndMeth=Simplest  InputSameDT=on  LockScale=on
  Bias1 : Bias  Bias=1
  Constant : Constant  Value=(pi/2) / (pi)  OutDataTypeStr=Inherit: Inherit via back propagation
  Divide1 : Product  Inputs=*/  OutDataTypeStr=fixdt(0,16,15)
  Divide2 : Product  Inputs=*/  OutDataTypeStr=fixdt(0,16,15)
  Gain : Gain  Gain=-1  OutDataTypeStr=Inherit: Same as input
  Logical Operator : Logic  Operator=XOR  AllPortsSameDT=off  OutDataTypeStr=boolean
  Relational Operator : RelationalOperator  Operator=<=  OutDataTypeStr=boolean
  Sum : Sum  Inputs=+-
  Switch{,1..3} (4 alike) : Switch  Criteria=u2 ~= 0
  abs : Subsystem
  abs1 : Subsystem
  angle : Outport
  wires:
  Switch1/1 -> Switch2/3, Gain/1
  Logical Operator/1 -> Switch2/2
  abs1/2(sign) -> Switch3/2, Logical Operator/2
  abs/2(sign) -> Logical Operator/1
  y/1 -> abs1/1(In3)
  abs1/1(abs) -> Divide1/2, Divide2/1, Relational Operator/2
  x/1 -> abs/1(In3)
  abs/1(abs) -> Divide2/2, Divide1/1, Relational Operator/1
  Sum/1 -> Switch1/3
  Constant/1 -> Sum/1
  1-D Lookup Table/1 -> Sum/2, Switch1/1
  Switch/1 -> 1-D Lookup Table/1
  Divide1/1 -> Switch/1
  Divide2/1 -> Switch/3
  Relational Operator/1 -> Switch1/2, Switch/2
  Switch2/1 -> Bias1/1, Switch3/1
  Switch3/1 -> angle/1
  Bias1/1 -> Switch3/3
  Gain/1 -> Switch2/1

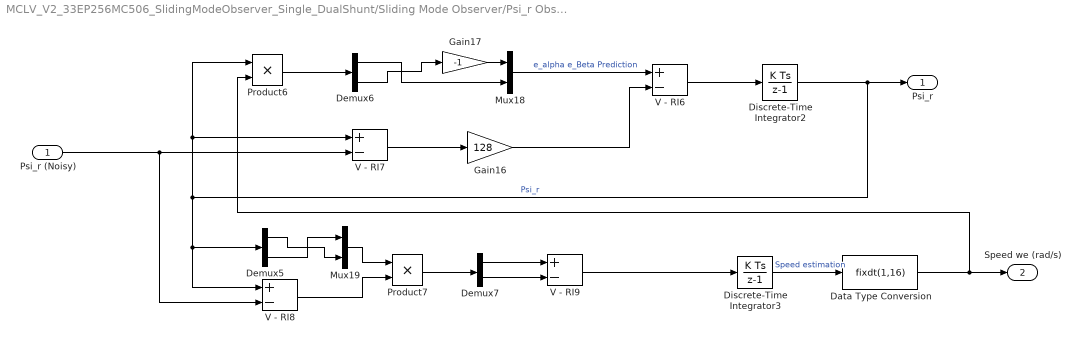
== system MCLV_V2_33EP256MC506_SlidingModeObserver_Single_DualShunt/Sliding Mode Observer/Psi_r Observer Speed Observer2 ==
  Psi_r (Noisy) : Inport
  Data Type Conversion : DataTypeConversion  OutMin=-5300 * 5 * (2*pi) / 60  OutMax=+5300 * 5 * (2*pi) / 60  OutDataTypeStr=fixdt(1,16)
  Demux5 : Demux  Outputs=2
  Demux6 : Demux  Outputs=2
  Demux7 : Demux  Outputs=2
  Discrete-Time Integrator2 : DiscreteIntegrator  gainval=1  SampleTime=-1  OutMin=-24  OutMax=24  OutDataTypeStr=fixdt(1,16)  UpperSaturationLimit=15  LowerSaturationLimit=-15  ICPrevOutput=DiscIntNeverNeededParam  ICPrevScaledInput=DiscIntNeverNeededParam
  Discrete-Time Integrator3 : DiscreteIntegrator  gainval=1000  SampleTime=-1  OutMin=-5300 * 5 * (2*pi) / 60  OutMax=5300 * 5 * (2*pi) / 60  OutDataTypeStr=fixdt(1,32)  RndMeth=Simplest  StateIdentifier=Speed  ICPrevOutput=DiscIntNeverNeededParam  ICPrevScaledInput=DiscIntNeverNeededParam
  Gain16 : Gain  Gain=128  OutMin=[-24*2*128]  OutMax=[24*2*128]  OutDataTypeStr=fixdt(1,16)
  Gain17 : Gain  Gain=-1  OutDataTypeStr=Inherit: Same as input
  Mux18 : Mux  Inputs=2
  Mux19 : Mux  Inputs=2
  Product6 : Product  OutDataTypeStr=fixdt(1,32,12)  SaturateOnIntegerOverflow=on  RndMeth=Zero
  Product7 : Product  OutMin=[-24*24]  OutMax=24*24  OutDataTypeStr=fixdt(1,16)  RndMeth=Simplest  SaturateOnIntegerOverflow=on
  V - RI6 : Sum  Inputs=+-  OutDataTypeStr=Inherit: Same as accumulator
  V - RI7 : Sum  Inputs=+-  OutMin=[-24*2]  OutMax=[24*2]  OutDataTypeStr=fixdt(1,16)
  V - RI8 : Sum  Inputs=+-  OutDataTypeStr=Inherit: Same as accumulator  RndMeth=Simplest  SaturateOnIntegerOverflow=on
  V - RI9 : Sum  Inputs=+-  OutMin=[-24*24*2]  OutMax=[-24*24*2]  OutDataTypeStr=fixdt(1,16)  RndMeth=Simplest  SaturateOnIntegerOverflow=on  InputSameDT=on
  Psi_r : Outport
  Speed we (rad/s) : Outport  Port=2
  wires:
  Gain16/1 -> V - RI6/2
  Discrete-Time Integrator2/1 -> Demux5/1, V - RI8/1, V - RI7/1, Product6/1, Psi_r/1  "Psi_r"
  Demux5/1 -> Mux19/2
  Demux6/2 -> Gain17/1
  Data Type Conversion/1 -> Speed we (rad/s)/1, Product6/2
  Psi_r (Noisy)/1 -> V - RI7/2, V - RI8/2
  Demux6/1 -> Mux18/2
  Discrete-Time Integrator3/1 -> Data Type Conversion/1  "Speed estimation"
  Gain17/1 -> Mux18/1
  Product6/1 -> Demux6/1
  Demux7/2 -> V - RI9/2
  Demux7/1 -> V - RI9/1
  Product7/1 -> Demux7/1
  V - RI8/1 -> Product7/2
  Mux19/1 -> Product7/1
  Demux5/2 -> Mux19/1
  Mux18/1 -> V - RI6/1  "e_alpha e_Beta Prediction"
  V - RI7/1 -> Gain16/1
  V - RI6/1 -> Discrete-Time Integrator2/1
  V - RI9/1 -> Discrete-Time Integrator3/1

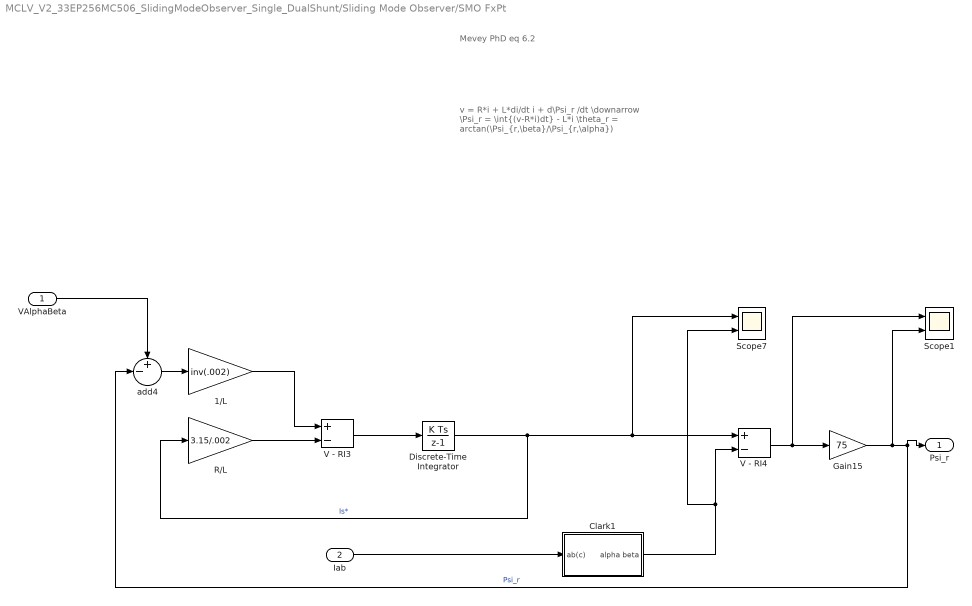
== system MCLV_V2_33EP256MC506_SlidingModeObserver_Single_DualShunt/Sliding Mode Observer/SMO FxPt ==
  note: Mevey PhD eq 6.2
  note: v = R*i + L*di/dt i + d\Psi_r /dt
      | \downarrow
      | \Psi_r = \int{(v-R*i)dt} - L*i
      | \theta_r = arctan(\Psi_{r,\beta}/\Psi_{r,\alpha})
  VAlphaBeta : Inport
  Iab : Inport  Port=2
  1/L : Gain  Gain=inv(.002)  OutMin=[-24] * inv(.002) *2  OutMax=[24] * inv(.002) *2  OutDataTypeStr=fixdt(1,16)
  Clark1 : Subsystem
  Discrete-Time Integrator : DiscreteIntegrator  SampleTime=-1  OutMin=[-4.4]  OutMax=[4.4]  OutDataTypeStr=fixdt(1,16)  ICPrevOutput=DiscIntNeverNeededParam  ICPrevScaledInput=DiscIntNeverNeededParam
  Gain15 : Gain  Gain=75  OutMin=[-24]  OutMax=[24]  OutDataTypeStr=fixdt(1,16)  SaturateOnIntegerOverflow=on
  R/L : Gain  Gain=3.15/.002  OutMin=[-4.4] * 3.15/.002  OutMax=[4.4] * 3.15/.002  OutDataTypeStr=fixdt(1,16)
  Scope1 : Scope  NumInputPorts=2
  Scope7 : Scope  NumInputPorts=2
  V - RI3 : Sum  Inputs=+-  OutDataTypeStr=Inherit: Same as accumulator
  V - RI4 : Sum  Inputs=+-  OutDataTypeStr=Inherit: Same as accumulator
  add4 : Sum  Inputs=+-|  OutDataTypeStr=Inherit: Same as accumulator  SaturateOnIntegerOverflow=on
  Psi_r : Outport
  wires:
  1/L/1 -> V - RI3/1
  R/L/1 -> V - RI3/2
  add4/1 -> 1/L/1
  VAlphaBeta/1 -> add4/1
  V - RI3/1 -> Discrete-Time Integrator/1
  Discrete-Time Integrator/1 -> V - RI4/1, Scope7/1, R/L/1  "Is*"
  V - RI4/1 -> Scope1/1, Gain15/1
  Iab/1 -> Clark1/1(ab(c))
  Clark1/1(alpha beta) -> V - RI4/2, Scope7/2
  Gain15/1 -> Scope1/2, add4/2, Psi_r/1  "Psi_r"

== system MCLV_V2_33EP256MC506_SlidingModeObserver_Single_DualShunt/Sliding Mode Observer/Atan x1/abs ==
  In3 : Inport
  Compare To Zero : simulink/Logic and Bit Operations/Compare To Zero  relop=>=  OutDataTypeStr=boolean
  Gain : Gain  Gain=-1  OutDataTypeStr=Inherit: Same as input
  Switch2 : Switch  Criteria=u2 ~= 0
  abs : Outport
  sign : Outport  Port=2
  wires:
  Compare To Zero/1 -> Switch2/2, sign/1
  In3/1 -> Compare To Zero/1, Switch2/1, Gain/1
  Gain/1 -> Switch2/3
  Switch2/1 -> abs/1

== system MCLV_V2_33EP256MC506_SlidingModeObserver_Single_DualShunt/Sliding Mode Observer/Atan x1/abs1 ==
  In3 : Inport
  Compare To Zero : simulink/Logic and Bit Operations/Compare To Zero  relop=>=  OutDataTypeStr=boolean
  Gain : Gain  Gain=-1  OutDataTypeStr=Inherit: Same as input
  Switch2 : Switch  Criteria=u2 ~= 0
  abs : Outport
  sign : Outport  Port=2
  wires:
  Switch2/1 -> abs/1
  Gain/1 -> Switch2/3
  In3/1 -> Gain/1, Switch2/1, Compare To Zero/1
  Compare To Zero/1 -> sign/1, Switch2/2

== system MCLV_V2_33EP256MC506_SlidingModeObserver_Single_DualShunt/Sliding Mode Observer/Atan x2/abs ==
  In3 : Inport
  Compare To Zero : simulink/Logic and Bit Operations/Compare To Zero  relop=>=  OutDataTypeStr=boolean
  Gain : Gain  Gain=-1  OutDataTypeStr=Inherit: Same as input
  Switch2 : Switch  Criteria=u2 ~= 0
  abs : Outport
  sign : Outport  Port=2
  wires:
  Switch2/1 -> abs/1
  Gain/1 -> Switch2/3
  In3/1 -> Gain/1, Switch2/1, Compare To Zero/1
  Compare To Zero/1 -> sign/1, Switch2/2

== system MCLV_V2_33EP256MC506_SlidingModeObserver_Single_DualShunt/Sliding Mode Observer/Atan x2/abs1 ==
  In3 : Inport
  Compare To Zero : simulink/Logic and Bit Operations/Compare To Zero  relop=>=  OutDataTypeStr=boolean
  Gain : Gain  Gain=-1  OutDataTypeStr=Inherit: Same as input
  Switch2 : Switch  Criteria=u2 ~= 0
  abs : Outport
  sign : Outport  Port=2
  wires:
  Compare To Zero/1 -> Switch2/2, sign/1
  In3/1 -> Compare To Zero/1, Switch2/1, Gain/1
  Gain/1 -> Switch2/3
  Switch2/1 -> abs/1

== system MCLV_V2_33EP256MC506_SlidingModeObserver_Single_DualShunt/Sliding Mode Observer/SMO FxPt/Clark1 ==
  note: Input is a vector of 3 elements, 3rd element is not beeing used
  note: k = 2/3 : invariant Magnitude
  ab(c) : Inport
  Clarke1 : Product  Multiplication=Matrix(*)  OutMin=[-4.4]  OutMax=[4.4]  OutDataTypeStr=fixdt(1,16)  SaturateOnIntegerOverflow=on  RndMeth=Zero
  Constant Magnitude : Constant  Value=[1 0 ; 1/sqrt(3) 2/sqrt(3) ];  OutDataTypeStr=fixdt(1,16)
  alpha beta : Outport
  wires:
  ab(c)/1 -> Clarke1/2
  Clarke1/1 -> alpha beta/1
  Constant Magnitude/1 -> Clarke1/1
